simulink model "rubik_cube"  (R2022b)
settings: Solver=FixedStepDiscrete  StartTime=0.0  StopTime=10000.0  FixedStep=0.1  RelTol=1e-3
InitFcn:
  | mbd_s32k_consistency_checks(bdroot(gcs));
undefined symbols (not defined in the file or in its folder): LQFP
libraries: mbd_s32k1xx_ec_toolbox x5
settings Model: Creator=leona  LastModifiedBy=leona
settings SolverCC: ZeroCrossControl=DisableAll
settings DataIOCC: SaveOutput=off  SaveState=on  SaveTime=off
settings OptimizationCC: DefaultParameterBehavior=Inlined  EnhancedBackFolding=on  PassReuseOutputArgsAs=Individual arguments  ZeroExternalMemoryAtStartup=off  ZeroInternalMemoryAtStartup=off  OptimizeBlockOrder=speed  DifferentSizesBufferReuse=on  OptimizationCustomize=off  EfficientTunableParamExpr=on
settings DebuggingCC: InheritedTsInSrcMsg=none  SingleTaskRateTransMsg=error  ParameterTunabilityLossMsg=error  UnconnectedInputMsg=error  UnconnectedOutputMsg=error  UnconnectedLineMsg=error  UnknownTsInhSupMsg=error
settings HardwareCC: ProdBitPerPointer=32  ProdBitPerSizeT=32  ProdBitPerPtrDiffT=32  ProdLargestAtomicInteger=Long  ProdLargestAtomicFloat=Double  ProdWordSize=32  ProdHWDeviceType=ARM Compatible->ARM Cortex
settings ModelReferenceCC: ModelReferenceNumInstancesAllowed=Single
settings SFSimCC: MATLABDynamicMemAlloc=off
settings RTWCC: Description=Model Based Design Toolbox S32K1xx Code Generation Target  SystemTargetFile=mbd_s32k.tlc  MakeCommand=mbd_s32k_make_rtw COPY_MDLREF_INCLUDES=0  TemplateMakefile=mbd_s32k.tmf
settings CodeAppCC: ForceParamTrailComments=on  IgnoreCustomStorageClasses=off  OperatorAnnotations=on  SimulinkDataObjDesc=on  SFDataObjDesc=on  InsertBlockDesc=on
settings STFCustomTargetCC: TargetLangStandard=C99 (ISO)  MultiwordLength=256  ERTCustomFileBanners=on  SupportContinuousTime=off  SupportNonInlinedSFcns=off  RemoveResetFunc=on  MATLABClassNameForMDSCustomization=Simulink.SoftwareTarget.ERTCustomization  SystemTargetFile=mbd_s32k.tlc
settings ERTTargetCC: TargetLangStandard=C99 (ISO)  ParMdlRefBuildCompliant=off  CompOptLevelCompliant=off  ConcurrentExecutionCompliant=off  CombineOutputUpdateFcns=off  ModelStepFunctionPrototypeControlCompliant=off  CPPClassGenCompliant=off  UseToolchainInfoCompliant=off  InlinedParameterPlacement=NonHierarchical  ERTSrcFileBannerTemplate=mbd_ert_code_template.cgt  ERTHdrFileBannerTemplate=mbd_ert_code_template.cgt  ERTDataSrcFileTemplate=mbd_ert_code_template.cgt  ERTDataHdrFileTemplate=mbd_ert_code_template.cgt  ERTCustomFileTemplate=example_file_process.tlc

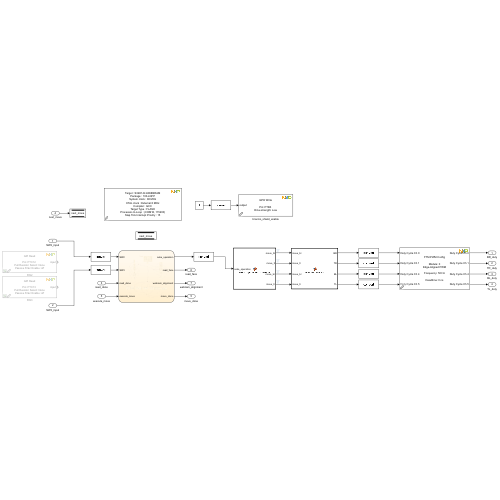
[thumbnail: Simulink's stored preview of the top-level diagram]
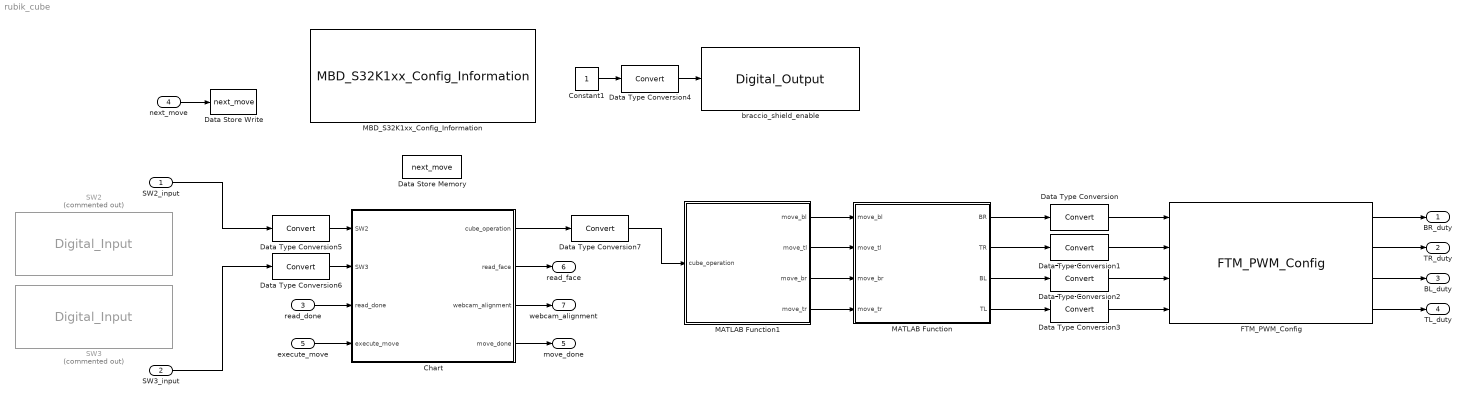
== system rubik_cube ==
  SW2_input : Inport
  SW3_input : Inport  Port=2
  read_done : Inport  Port=3
  next_move : Inport  Port=4
  execute_move : Inport  Port=5
  Chart : Stateflow chart  TreatAsAtomicUnit=on
  Constant1 : Constant
  Data Store Memory : DataStoreMemory  DataStoreName=next_move  WriteAfterWriteMsg=warning  InitialValue=uint8(zeros(1,2))  ShowAdditionalParam=off  OutDataTypeStr=uint8
  Data Store Write : DataStoreWrite  DataStoreName=next_move  IndexOptions=Index vector (dialog)  Indices=1  OutputSizes=1
  Data Type Conversion{,1..7} (8 alike) : DataTypeConversion  SaturateOnIntegerOverflow=off  RndMeth=Floor
  FTM_PWM_Config : mbd_s32k1xx_ec_toolbox/Motor Control Blocks/FTM Blocks/FTM_PWM_Config  ftmModule=0  ftmMode=Edge-Aligned PWM  ftmSourceClock=80 MHz  swcontrol_enable=off  chan0En=on  chan0Type=Independent  chan2En=off  chan2Type=Independent  chan4En=on  chan4Type=Independent  chan6En=off  chan6Type=Independent  ftmPwmUnits=Hz  outFrequency=50  ftmPeriod=25000  ftmPrescaler=Divide by 64  deadtimeUnits=Nanoseconds  deadtimeNs=0  deadtimeTicks=0  deadtimePrescaler=Divide by 1  dutyCycleCh0=0.03  dutyCycleCh1=0.125  dutyCycleCh2=0.025  dutyCycleCh3=0.025  dutyCycleCh4=0.025  dutyCycleCh5=0.025  dutyCycleCh6=0.25  dutyCycleCh7=0.25  dutyCycleSim=on  startAfterInit=on  showAdvOpt=on  pinFtmCh0=PTD15: [FTM0_CH0 | FTM Channel]  pinFtmCh1=PTD16: [FTM0_CH1 | FTM Channel]  pinPolCh0=Active High  pinPolCh1=Active High  outputComplem0=Main duplicated  outputLevel0=Low  outputLevel1=Low  pinFtmCh2=PTB14: [FTM0_CH2 | FTM Channel]  pinFtmCh3=PTC3: [FTM0_CH3 | FTM Channel]  pinPolCh2=Active High  pinPolCh3=Active High  outputComplem2=Main duplicated  outputLevel2=Low  outputLevel3=Low  pinFtmCh4=PTB4: [FTM0_CH4 | FTM Channel]  pinFtmCh5=PTB5: [FTM0_CH5 | FTM Channel]  pinPolCh4=Active High  pinPolCh5=Active High  outputComplem4=Main duplicated  outputLevel4=Low  outputLevel5=Low  pinFtmCh6=PTE8: [FTM0_CH6 | FTM Channel]  pinFtmCh7=None  pinPolCh6=Active High  pinPolCh7=Active High  outputComplem6=Main duplicated  outputLevel6=Low  outputLevel7=Low  initTrigger=off  chTrigger0=off  chTrigger1=off  chTrigger2=off  chTrigger3=off  chTrigger4=off  chTrigger5=off  chTrigger6=off  chTrigger7=off  mcuTargetUpdate=on  pwmSyncTrg=Software trigger  pwmSyncHwRouting=TRGMUX_FTM7  pwmSyncTrg0=off  pwmSyncTrg1=off  pwmSyncTrg2=off  pwmSyncAutoClear=on  pwmSyncMinLoad=on  pwmSyncMaxLoad=on  pwmSyncInvert=System Clock  pwmSyncOutControl=System Clock  pwmSyncOutMask=System Clock  pwmSyncCounterInitial=System Clock  pwmSyncPoints=Update now  reloadEnable=off  reloadPriority=15  reloadHalfCycle=off  reloadHCR=0  reloadFrequency=0  chnMatch0=off  chnMatch1=off  chnMatch2=off  chnMatch3=off  chnMatch4=off  chnMatch5=off  chnMatch6=off  chnMatch7=off  pwmFaultProtection=off  pwmFaultInterrupt=off  pwmFaultClearing=Fault control disabled  pwmFaultPinState=Safe Value  pwmFaultFilterValue=0  pwmFaultPriority=15  fault_disen_0=off  fault_filter_0=off  fault_polarity_0=Active High  fault_disen_1=off  fault_filter_1=off  fault_polarity_1=Active high  fault_disen_2=off  fault_filter_2=off  fault_polarity_2=Active high  fault_disen_3=off  fault_filter_3=off  fault_polarity_3=Active high  fault_pin_0=None  fault_pin_1=None  fault_pin_2=None  fault_pin_3=None
  MATLAB Function : MATLAB Function  TreatAsAtomicUnit=on
  MATLAB Function1 : MATLAB Function  TreatAsAtomicUnit=on
  MBD_S32K1xx_Config_Information : mbd_s32k1xx_ec_toolbox/MBD_S32K1xx_Config_Information  mbdt_ver=0  disp_str=|  config_params=[]  mcu_target_name=S32K144  mcu_target_package=100-LQFP  mcu_target_sram_size=48KB  mcu_system_clock_freq=80  mcu_xtal_freq=External 8  mcu_steptick_timer=LPIT Channel 0  mcu_steptick_prio=15  ds_import_enable=on  target_compiler=GCC  target_memory=FLASH  gcc_target_compile_opts=-mthumb -mfloat-abi=hard -mfpu=fpv4-sp-d16 -O1 -g -gstrict-dwarf  gcc_target_assemble_opts=-mthumb -mfloat-abi=hard -mfpu=fpv4-sp-d16 -g  gcc_target_link_opts=-mthumb -mfloat-abi=hard -mfpu=fpv4-sp-d16  gcc_target_default_lcf=on  gcc_target_user_lcf=S32K144_48_flash.ld  ghs_target_compile_opts=-cpu=cortexm4f -thumb -fpu=vfpv4_d16 -fsingle -Ogeneral -Wundef -Wimplicit-int -Wshadow -Wtrigraphs --no_commons --gnu_asm -gnu99 -gdwarf-2 -G  ghs_target_assemble_opts=-cpu=cortexm4f -fpu=vfpv4_d16  ghs_target_link_opts=-cpu=cortexm4f -thumb -fpu=vfpv4_d16  ghs_target_default_lcf=on  ghs_target_user_lcf=S32K144_48_flash.ld  iar_target_compile_opts=--cpu=Cortex-M4F --thumb --fpu=VFPv4_sp -Ol -e --debug --dlib_config normal  iar_target_assemble_opts=--cpu Cortex-M4F --thumb --fpu VFPv4_sp  iar_target_link_opts=--no_exceptions --vfe --inline  iar_target_default_lcf=on  iar_target_user_lcf=S32K144_48_flash.icf  pil_download_enable=on  rbl_download_enable=on  rbl_start_delay=5000  rbl_download_interface=OpenSDA  rbl_restart_request=off  rbl_com_port=Custom  rbl_com_port_custom=COM18  pil_download_rate=115200  pil_download_rate_custom=115200  pil_opensda_drive=F: EVB-S32K144  pil_opensda_drive_custom=D  jtag_interface=OpenSDA Embedded Debug  jlink_default_path=on  jlink_user_path=C:\Program Files\SEGGER\JLink\  pil_uart_instance=1  pil_uart_rx=PTC6: [LPUART1_RX | Receive]  pil_uart_tx=PTC7: [LPUART1_TX | Transmit]  FTM_PWM_PcrCheckEnDis=on  FTM_Input_Edge_Inputs_PcrCheckEnDis=on  FTM_Dual_Edge_Inputs_PcrCheckEnDis=on  FTM_Quadrature_Inputs_PcrCheckEnDis=on  FTM_Hall_Sensor_Inputs_PcrCheckEnDis=on  LPTMR_PcrCheckEnDis=on  PIT_PcrCheckEnDis=on  RTC_PcrCheckEnDis=on  FlexCAN_PcrCheckEnDis=on  LIN_PcrCheckEnDis=on  FlexIO_PcrCheckEnDis=on  LPI2C_PcrCheckEnDis=on  LPSPI_PcrCheckEnDis=on  LPUART_PcrCheckEnDis=on  CMP_PcrCheckEnDis=on  GPIO_OutputPcrCheckEnDis=on  GPIO_InputPcrCheckEnDis=on  SBC_PcrCheckEnDis=on  BMS_PcrCheckEnDis=on  AMMCLIB_PcrCheckEnDis=on  FM_PcrCheckEnDis=on  Profile_PcrCheckEnDis=on  ConfigParams_PcrCheckEnDis=on  ModelRef_PcrCheckEnDis=on  PDB0_PcrCheckEnDis=on  CSEc_PcrCheckEnDis=on  eDMA_PcrCheckEnDis=on  FLASH_PcrCheckEnDis=on  ADC_PcrCheckEnDis=on  WDOG_PcrCheckEnDis=on
      | Target : S32K144-64KB_SRAM
      | Package : 100-pin
      | System clock : 80 MHz
      | XTAL clock : External 8 MHz
      | Compiler : IAR
      | Target Type : FLASH
      | Download Code after build : off
      | Step Tick Interrupt Priority : 15
  SW2 : mbd_s32k1xx_ec_toolbox/GPIO Blocks/Digital_Input  Commented=on  gpio_pin=PTC12: [PTC12 | Port C I/O]  pull_resistor=None  passive_filter=off
  SW3 : mbd_s32k1xx_ec_toolbox/GPIO Blocks/Digital_Input  Commented=on  gpio_pin=PTC13: [PTC13 | Port C I/O]  pull_resistor=None  passive_filter=off
  braccio_shield_enable : mbd_s32k1xx_ec_toolbox/GPIO Blocks/Digital_Output  gpio_pin=PTB3: [PTB3 | Port B I/O]  init_val=Low  drive_strength=Low
  BR_duty : Outport
  TR_duty : Outport  Port=2
  BL_duty : Outport  Port=3
  TL_duty : Outport  Port=4
  move_done : Outport  Port=5
  read_face : Outport  Port=6
  webcam_alignment : Outport  Port=7
  wires:
  Data Type Conversion2/1 -> FTM_PWM_Config/3
  MATLAB Function1/3(move_br) -> MATLAB Function/3(move_br)
  FTM_PWM_Config/1 -> BR_duty/1
  MATLAB Function/4(TL) -> Data Type Conversion3/1
  FTM_PWM_Config/2 -> TR_duty/1
  Data Type Conversion5/1 -> Chart/1(SW2)
  Data Type Conversion4/1 -> braccio_shield_enable/1
  MATLAB Function/3(BL) -> Data Type Conversion2/1
  Chart/1(cube_operation) -> Data Type Conversion7/1
  Constant1/1 -> Data Type Conversion4/1
  MATLAB Function/1(BR) -> Data Type Conversion/1
  MATLAB Function1/1(move_bl) -> MATLAB Function/1(move_bl)
  FTM_PWM_Config/4 -> TL_duty/1
  Data Type Conversion7/1 -> MATLAB Function1/1(cube_operation)
  FTM_PWM_Config/3 -> BL_duty/1
  Data Type Conversion3/1 -> FTM_PWM_Config/4
  MATLAB Function/2(TR) -> Data Type Conversion1/1
  Data Type Conversion6/1 -> Chart/2(SW3)
  Data Type Conversion1/1 -> FTM_PWM_Config/2
  MATLAB Function1/4(move_tr) -> MATLAB Function/4(move_tr)
  Data Type Conversion/1 -> FTM_PWM_Config/1
  MATLAB Function1/2(move_tl) -> MATLAB Function/2(move_tl)
  SW2_input/1 -> Data Type Conversion5/1
  SW3_input/1 -> Data Type Conversion6/1
  Chart/2(read_face) -> read_face/1
  Chart/3(webcam_alignment) -> webcam_alignment/1
  Chart/4(move_done) -> move_done/1
  read_done/1 -> Chart/3(read_done)
  execute_move/1 -> Chart/4(execute_move)
  next_move/1 -> Data Store Write/1

== matlab function rubik_cube/MATLAB Function1 ==
  data: cube_operation input; move_bl output; move_tl output; move_br output; move_tr output
function [move_bl, move_tl, move_br, move_tr] = cube_operation_decoder(cube_operation)
% This function takes as input the code for a cube operation and converts
% it as positions of the 4 servo motors. The operations must be a 4 digit
% unsigned integer, encoded as follows:
%   - first digit [0, 1]: open/close left grip;
%   - second digit [0, 1]: open/close right grip;
%   - third digit [0, 1, 2]: set left arm to 90/0/180 degrees
%   - fourth digit [0, 1, 2]: set right arm to 90/0/180 degress

x1 = int32(mod(cube_operation/1000, 10));
x2 = int32(mod(cube_operation/100, 10));
x3 = int32(mod(cube_operation/10, 10));
x4 = int32(mod(cube_operation, 10));

move_tl = x1;
move_tr = x2;
move_bl = x3;
move_br = x4;

== matlab function rubik_cube/MATLAB Function ==
  data: BR output; TR output; move_bl input; BL output; move_tl input; move_br input; move_tr input; TL output
function [BR, TR, BL, TL] = actuate_servos(move_bl, move_tl, move_br, move_tr)
% This function takes as input as specific number associated to a movement
% of the 4 servo motors (BL = Bottom Left, TL = Top Left, BR = Bottom Right,
% TR = Top Right) and it gives as output the 4 relative duty cycles needed to
% obtain that movement. 

min_duty = 0.025;
max_duty = 0.125;

duty_0_deg = min_duty;
duty_grip_open = min_duty + (max_duty-min_duty)/3;
duty_grip_closed = min_duty + (max_duty-min_duty)/9; 
duty_90_deg = min_duty + (max_duty-min_duty)/2;
duty_180_deg = max_duty;

switch (move_tl)
    case 0                  % Open left grip
        TL = duty_grip_open;
    case 1                  % Close left grip
        TL = duty_grip_closed;
    otherwise               % Open left grip
        TL = duty_grip_open;
end

switch (move_tr)
    case 0                  % Open right grip
        TR = duty_grip_open;
    case 1                  % Close right grip
        TR = duty_grip_closed;
    otherwise               % Open right grip
        TR = duty_grip_open;
end

switch (move_bl)
    case 0                  % Left arm straight
        BL = duty_90_deg;
    case 1                  % Left arm at 90° clockwise
        BL = duty_0_deg;
    case 2                  % Left arm at 90° counter-clockwise
        BL = duty_180_deg;
    otherwise
        BL = duty_90_deg;
end

switch (move_br)
    case 0                  % Right arm straight
        BR = duty_90_deg;
    case 1                  % Right arm at 90° clockwise
        BR = duty_0_deg;
    case 2                  % Right arm at 90° counter-clockwise
        BR = duty_180_deg;
    otherwise
        BR = duty_90_deg;
end

% Update current position of the motors
BL_last_move = move_bl;
TL_last_move = move_tl;
BR_last_move = move_br;
TR_last_move = move_tr;

== stateflow chart rubik_cube/Chart ==
  state read_cube
    en:
    webcam_alignment = 0;
    SW3_status = SW3;
    du:
    SW3_status = SW3;
    % Clear cube colors
    %cube = zeros(3, 3, 6);
    %read red
    %LTm
    %read blue
    %LTm
    %read orange
    %LTm
    %read green
    %RTm
    %LTm
    %read white
    %RTmm
    %LTmm
    %read yellow
    %RTm
    %LTm
    %RTp
    state read_red
      en:
      read_face = 1;
    state wait_red
      en:
      read_face = 0;
    state fase1
      en:
      cube_operation=1000
    state fase2
      en:
      cube_operation=1010
    state fase3
      en:
      cube_operation=1110
    state fase4
      en:
      cube_operation=0110
    state fase5
      en:
      cube_operation=0100
    state fase6
      en:
      cube_operation=1100
    state fase12
      en:
      cube_operation=1100
    state fase11
      en:
      cube_operation=0100
    state fase10
      en:
      cube_operation=0110
    state fase9
      en:
      cube_operation=1110
    state fase8
      en:
      cube_operation=1010
    state fase7
      en:
      cube_operation=1000
    state wait_blue
      en:
      read_face = 0;
    state read_blue
      en:
      read_face = 1;
    state read_orange
      en:
      read_face=1;
    state wait_orange
      en:
      read_face=0;
    state fase13
      en:
      cube_operation=1000
    state fase14
      en:
      cube_operation=1010
    state fase15
      en:
      cube_operation=1110
    state fase16
      en:
      cube_operation=0110
    state fase17
      en:
      cube_operation=0100
    state fase18
      en:
      cube_operation=1100
    state fase24
      en:
      cube_operation=1100
    state fase23
      en:
      cube_operation=1000
    state fase22
      en:
      cube_operation=1001
    state fase21
      en:
      cube_operation=1101
    state fase20
      en:
      cube_operation=0101
    state fase19
      en:
      cube_operation=0100
    state wait_green
      en:
      read_face=0;
    state read_green
      en:
      read_face=1;
    state fase27
      en:
      cube_operation=1110
    state fase25
      en:
      cube_operation=1000
    state fase26
      en:
      cube_operation=1010
    state fase28
      en:
      cube_operation=0110
    state fase29
      en:
      cube_operation=0100
    state fase30
      en:
      cube_operation=1100
    state read_white
      en:
      read_face=1;
    state wait_white
      en:
      read_face=0;
    state fase35
      en:
      cube_operation=1000
    state fase37
      en:
      cube_operation=0100
    state fase36
      en:
      cube_operation=1100
    state fase34
      en:
      cube_operation=1001
    state fase33
      en:
      cube_operation=1101
    state fase32
      en:
      cube_operation=0101
    state fase31
      en:
      cube_operation=0100
    state fase38
      en:
      cube_operation=0101
    state fase39
      en:
      cube_operation=1101
    state fase40
      en:
      cube_operation=1001
    state fase41
      en:
      cube_operation=1000
    state fase42
      en:
      cube_operation=1100
    state fase43
      en:
      cube_operation=1000
    state fase44
      en:
      cube_operation=1010
    state fase51
      en:
      cube_operation=1110
    state fase50
      en:
      cube_operation=1010
    state fase49
      en:
      cube_operation=1000
    state fase48
      en:
      cube_operation=1100
    state fase47
      en:
      cube_operation=0100
    state fase46
      en:
      cube_operation=0110
    state fase45
      en:
      cube_operation=1110
    state read_yellow
      en:
      read_face=1;
    state wait_yellow
      en:
      read_face=0;
    state fase55
      en:
      cube_operation=0100
    state fase56
      en:
      cube_operation=0101
    state fase57
      en:
      cube_operation=1101
    state fase52
      en:
      cube_operation=0110
    state fase54
      en:
      cube_operation=1100
    state fase53
      en:
      cube_operation=0100
    state fase58
      en:
      cube_operation=1001
    state fase63
      en:
      cube_operation=1110
    state fase64
      en:
      cube_operation=0110
    state fase62
      en:
      cube_operation=1010
    state fase61
      en:
      cube_operation=1000
    state fase60
      en:
      cube_operation=1100
    state fase59
      en:
      cube_operation=1000
    state fase65
      en:
      cube_operation=0100
    state fase66
      en:
      cube_operation=1100
    state fase67
      en:
      cube_operation=1000
    state fase68
      en:
      cube_operation=1001
    state fase69
      en:
      cube_operation=1101
    state fase70
      en:
      cube_operation=0101
    state fase71
      en:
      cube_operation=0100
    state fase72
      en:
      cube_operation=1100
    (default) -> read_red
    wait_red -> read_red [order 2] : [read_done==2]
    read_red -> wait_red
    wait_red -> read_cube.fase1 [order 1] : [read_done==1]
    read_cube.fase1 -> read_cube.fase2 : [SW3 == 1]
    read_cube.fase2 -> read_cube.fase3 : [after(delay_ms, msec)]
    read_cube.fase3 -> read_cube.fase4 : [after(delay_ms, msec)]
    read_cube.fase4 -> read_cube.fase5 : [after(delay_ms, msec)]
    read_cube.fase5 -> read_cube.fase6 : [after(delay_ms, msec)]
    read_cube.fase6 -> read_blue : [after(delay_ms, msec)]
    wait_blue -> read_blue [order 2] : [read_done==2]
    read_blue -> wait_blue
    read_cube.fase11 -> read_cube.fase12 : [after(delay_ms, msec)]
    read_cube.fase10 -> read_cube.fase11 : [after(delay_ms, msec)]
    read_cube.fase9 -> read_cube.fase10 : [after(delay_ms, msec)]
    read_cube.fase8 -> read_cube.fase9 : [after(delay_ms, msec)]
    read_cube.fase7 -> read_cube.fase8 : [SW3 == 1]
    wait_blue -> read_cube.fase7 [order 1] : [read_done==1]
    read_cube.fase12 -> read_orange : [after(delay_ms, msec)]
    wait_orange -> read_orange [order 1] : [read_done==2]
    read_orange -> wait_orange
    wait_orange -> read_cube.fase13 [order 2] : [read_done==1]
    read_cube.fase13 -> read_cube.fase14 : [SW3 == 1]
    read_cube.fase14 -> read_cube.fase15 : [after(delay_ms, msec)]
    read_cube.fase15 -> read_cube.fase16 : [after(delay_ms, msec)]
    read_cube.fase16 -> fase17 : [after(delay_ms, msec)]
    fase17 -> fase18 : [after(delay_ms, msec)]
    fase18 -> read_green : [after(delay_ms, msec)]
    read_green -> wait_green
    fase23 -> fase24 : [after(delay_ms, msec)]
    fase22 -> fase23 : [after(delay_ms, msec)]
    fase21 -> fase22 : [after(delay_ms, msec)]
    fase20 -> fase21 : [after(delay_ms, msec)]
    fase19 -> fase20 : [SW3 == 1]
    wait_green -> fase19 [order 1] : [read_done==1]
    wait_green -> read_green [order 2] : [read_done==2]
    fase24 -> fase25 : [after(delay_ms, msec)]
    read_white -> wait_white
    fase26 -> fase27 : [after(delay_ms, msec)]
    fase27 -> fase28 : [after(delay_ms, msec)]
    fase25 -> fase26 : [after(delay_ms, msec)]
    fase28 -> fase29 : [after(delay_ms, msec)]
    fase29 -> fase30 : [after(delay_ms, msec)]
    wait_white -> read_white [order 2] : [read_done==2]
    fase30 -> read_white : [after(delay_ms, msec)]
    wait_white -> fase31 [order 1] : [read_done==1]
    fase35 -> fase36 : [after(delay_ms, msec)]
    fase34 -> fase35 : [[after(delay_ms, msec)]]
    fase36 -> fase37 : [after(delay_ms, msec)]
    fase33 -> fase34 : [after(delay_ms, msec)]
    fase32 -> fase33 : [after(delay_ms, msec)]
    fase31 -> fase32 : [SW3 == 1]
    fase37 -> fase38 : [after(delay_ms, msec)]
    fase39 -> fase40 : [after(delay_ms, msec)]
    fase38 -> fase39 : [after(delay_ms, msec)]
    fase40 -> fase41 : [after(delay_ms, msec)]
    fase41 -> fase42 : [after(delay_ms, msec)]
    fase42 -> fase43 : [after(delay_ms, msec)]
    fase43 -> fase44 : [after(delay_ms, msec)]
    fase44 -> fase45 : [after(delay_ms, msec)]
    fase49 -> fase50 : [after(delay_ms, msec)]
    fase48 -> fase49 : [after(delay_ms, msec)]
    fase46 -> fase47 : [after(delay_ms, msec)]
    fase45 -> fase46 : [after(delay_ms, msec)]
    fase50 -> fase51 : [after(delay_ms, msec)]
    fase47 -> fase48 : [after(delay_ms, msec)]
    fase51 -> fase52 : [after(delay_ms, msec)]
    fase56 -> fase57 : [after(delay_ms, msec)]
    fase54 -> read_yellow : [after(delay_ms, msec)]
    fase55 -> fase56 : [SW3 == 1]
    read_yellow -> wait_yellow
    wait_yellow -> fase55 [order 2] : [read_done==1]
    fase52 -> fase53 : [after(delay_ms, msec)]
    fase53 -> fase54 : [after(delay_ms, msec)]
    wait_yellow -> read_yellow [order 1] : [read_done==2]
    fase57 -> fase58 : [after(delay_ms, msec)]
    fase62 -> fase63 : [after(delay_ms, msec)]
    fase61 -> fase62 : [after(delay_ms, msec)]
    fase60 -> fase61 : [after(delay_ms, msec)]
    fase59 -> fase60 : [after(delay_ms, msec)]
    fase63 -> fase64 : [after(delay_ms, msec)]
    fase58 -> fase59 : [after(delay_ms, msec)]
    fase64 -> fase65 : [after(delay_ms, msec)]
    fase65 -> fase66 : [after(delay_ms, msec)]
    fase66 -> fase67 : [after(delay_ms, msec)]
    fase67 -> fase68 : [after(delay_ms, msec)]
    fase68 -> fase69 : [after(delay_ms, msec)]
    fase69 -> fase70 : [after(delay_ms, msec)]
    fase70 -> fase71 : [after(delay_ms, msec)]
    fase71 -> fase72 : [after(delay_ms, msec)]
  state webcam_alignment
    en:
    SW2_status = SW2;
    SW3_status = SW3;
    cube_operation=1100;
    webcam_alignment = 1;
    du:
    SW2_status=SW2;
    SW3_status=SW3;
  state wait_cube
    en:
    SW2_status = SW2;
    cube_operation=0100;
    move_done = 1;
    du:
    SW2_status=SW2;
  state D
    en:
    %LMp
    state fase1 %LMp
      en:
      cube_operation=0100;
    state fase2
      en:
      cube_operation=0110;
    state fase3
      en:
      cube_operation=1110;
    state fase4
      en:
      cube_operation=1100;
    (default) -> fase1 %LMp
    fase1 %LMp -> D.fase2 : [after(delay_ms,msec)]
    D.fase2 -> D.fase3 : [after(delay_ms,msec)]
    D.fase3 -> D.fase4 : [after(delay_ms,msec)]
  state Fi
    en:
    %LTpp
    %RMm
    state fase1
      en:
      cube_operation=0100;
    state fase1bis
      en:
      cube_operation=0110;
    state fase2
      en:
      cube_operation=1110;
    state fase4
      en:
      cube_operation=1120;
    state fase3bis
      en:
      cube_operation=1020;
    state fase3
      en:
      cube_operation=1010;
    state fase5bis
      en:
      cube_operation=0100;
    state fase6
      en:
      cube_operation=1100
    state fase5
      en:
      cube_operation=0120;
    state fase8bis
      en:
      cube_operation=1000;
    state fase8
      en:
      cube_operation=1001;
    state fase7 %RMm
      en:
      cube_operation=1101;
    state fase9
      en:
      cube_operation=1100;
    (default) -> Fi.fase1
    Fi.fase1 -> Fi.fase1bis : [after(delay_ms,msec)]
    Fi.fase1bis -> Fi.fase2 : [after(delay_ms,msec)]
    Fi.fase2 -> Fi.fase3 : [after(delay_ms,msec)]
    Fi.fase3bis -> Fi.fase4 : [after(delay_ms,msec)]
    Fi.fase3 -> Fi.fase3bis : [after(delay_ms,msec)]
    Fi.fase4 -> Fi.fase5 : [after(delay_ms,msec)]
    Fi.fase5bis -> Fi.fase6 : [after(delay_ms,msec)]
    Fi.fase5 -> Fi.fase5bis : [after(delay_ms,msec)]
    Fi.fase6 -> fase7 %RMm : [after(delay_ms,msec)]
    fase7 %RMm -> Fi.fase8 : [after(delay_ms,msec)]
    Fi.fase8 -> fase8bis : [after(delay_ms,msec)]
    fase8bis -> Fi.fase9 : [after(delay_ms,msec)]
  state solve_cube
    en:
    move_done = 1;
    ex:
    move_done = 0;
  state D2
    en:
    %LMpp
    state fase1 %LMpp
      en:
      cube_operation=0100;
    state fase2
      en:
      cube_operation=0110;
    state fase4
      en:
      cube_operation=1120;
    state fase3
      en:
      cube_operation=1110;
    state fase6
      en:
      cube_operation=0100;
    state fase5
      en:
      cube_operation=0120;
    state fase7
      en:
      cube_operation=1100;
    (default) -> fase1 %LMpp
    fase1 %LMpp -> D2.fase2 : [after(delay_ms,msec)]
    D2.fase2 -> D2.fase3 : [after(delay_ms,msec)]
    D2.fase3 -> D2.fase4 : [after(delay_ms,msec)]
    D2.fase4 -> D2.fase5 : [after(delay_ms,msec)]
    D2.fase5 -> D2.fase6 : [after(delay_ms,msec)]
    D2.fase6 -> D2.fase7 : [after(delay_ms,msec)]
  state F
    en:
    %LTpp
    %RMp
    state fase1
      en:
      cube_operation=0100;
    state fase1bis
      en:
      cube_operation=0110;
    state fase2
      en:
      cube_operation=1110;
    state fase4
      en:
      cube_operation=1120;
    state fase3bis
      en:
      cube_operation=1020;
    state fase3
      en:
      cube_operation=1010;
    state fase5bis
      en:
      cube_operation=0100;
    state fase6
      en:
      cube_operation=1100
    state fase5
      en:
      cube_operation=0120;
    state fase8
      en:
      cube_operation=1101;
    state fase7bis
      en:
      cube_operation=1001;
    state fase7 %RMp
      en:
      cube_operation=1000;
    state fase9
      en:
      cube_operation=1100;
    F.fase1 -> F.fase1bis : [after(delay_ms,msec)]
    F.fase1bis -> F.fase2 : [after(delay_ms,msec)]
    (default) -> F.fase1
    F.fase2 -> F.fase3 : [after(delay_ms,msec)]
    F.fase3bis -> F.fase4 : [after(delay_ms,msec)]
    F.fase3 -> F.fase3bis : [after(delay_ms,msec)]
    F.fase4 -> F.fase5 : [after(delay_ms,msec)]
    F.fase5bis -> F.fase6 : [after(delay_ms,msec)]
    F.fase5 -> F.fase5bis : [after(delay_ms,msec)]
    F.fase6 -> fase7 %RMp : [after(delay_ms,msec)]
    fase7 %RMp -> F.fase7bis : [after(delay_ms,msec)]
    F.fase7bis -> F.fase8 : [after(delay_ms,msec)]
    F.fase8 -> F.fase9 : [after(delay_ms,msec)]
  state Di
    en:
    %LMm
    state fase1 %LMm
      en:
      cube_operation=1110;
    state fase2
      en:
      cube_operation=0110;
    state fase3
      en:
      cube_operation=0100;
    state fase4
      en:
      cube_operation=1100;
    (default) -> fase1 %LMm
    fase1 %LMm -> Di.fase2 : [after(delay_ms,msec)]
    Di.fase2 -> Di.fase3 : [after(delay_ms,msec)]
    Di.fase3 -> Di.fase4 : [after(delay_ms,msec)]
  state F2
    en:
    %LTpp
    %RMpp
    state fase1
      en:
      cube_operation=0100;
    state fase1bis
      en:
      cube_operation=0110;
    state fase2
      en:
      cube_operation=1110;
    state fase4
      en:
      cube_operation=1120;
    state fase3bis
      en:
      cube_operation=1020;
    state fase3
      en:
      cube_operation=1010;
    state fase5bis
      en:
      cube_operation=0100;
    state fase6
      en:
      cube_operation=1100
    state fase5
      en:
      cube_operation=0120;
    state fase12 %RMpp
      en:
      cube_operation=1000;
    state fase7bis
      en:
      cube_operation=1001;
    state fase9
      en:
      cube_operation=1102;
    state fase8
      en:
      cube_operation=1101;
    state fase10
      en:
      cube_operation=1002;
    state fase11
      en:
      cube_operation=1100;
    state fase10bis
      en:
      cube_operation=1000;
    F2.fase1 -> F2.fase1bis : [after(delay_ms,msec)]
    F2.fase1bis -> F2.fase2 : [after(delay_ms,msec)]
    (default) -> F2.fase1
    F2.fase2 -> F2.fase3 : [after(delay_ms,msec)]
    F2.fase3bis -> F2.fase4 : [after(delay_ms,msec)]
    F2.fase3 -> F2.fase3bis : [after(delay_ms,msec)]
    F2.fase4 -> F2.fase5 : [after(delay_ms,msec)]
    F2.fase5bis -> F2.fase6 : [after(delay_ms,msec)]
    F2.fase5 -> F2.fase5bis : [after(delay_ms,msec)]
    F2.fase6 -> fase12 %RMpp : [after(delay_ms,msec)]
    fase12 %RMpp -> F2.fase7bis : [after(delay_ms,msec)]
    F2.fase7bis -> F2.fase8 : [after(delay_ms,msec)]
    F2.fase9 -> F2.fase10 : [after(delay_ms,msec)]
    F2.fase8 -> F2.fase9 : [after(delay_ms,msec)]
    F2.fase10 -> fase10bis : [after(delay_ms,msec)]
    fase10bis -> F2.fase11 : [after(delay_ms,msec)]
  state B
    en:
    %RMp
    state fase1 %RMp
      en:
      cube_operation=1000;
    state fase2
      en:
      cube_operation=1001;
    state fase3
      en:
      cube_operation=1101;
    state fase4
      en:
      cube_operation=1100;
    (default) -> fase1 %RMp
    fase1 %RMp -> B.fase2 : [after(delay_ms,msec)]
    B.fase2 -> B.fase3 : [after(delay_ms,msec)]
    B.fase3 -> B.fase4 : [after(delay_ms,msec)]
  state U
    %RTpp
    %LMp
    state fase1 %RTpp
      en:
      cube_operation=1000;
    state fase2
      en:
      cube_operation=1001;
    state fase3
      en:
      cube_operation=1101;
    state fase6
      en:
      cube_operation=1102;
    state fase5
      en:
      cube_operation=0102;
    state fase4
      en:
      cube_operation=0101;
    state fase8
      en:
      cube_operation=1000;
    state fase9
      en:
      cube_operation=1100;
    state fase7
      en:
      cube_operation=1002;
    state fase12
      en:
      cube_operation=1110;
    state fase11
      en:
      cube_operation=0110;
    state fase10 %LMp
      en:
      cube_operation=0100;
    state fase13
      en:
      cube_operation=1100;
    (default) -> U.fase1 %RTpp
    U.fase2 -> U.fase3 : [after(delay_ms,msec)]
    U.fase1 %RTpp -> U.fase2 : [after(delay_ms,msec)]
    U.fase3 -> U.fase4 : [after(delay_ms,msec)]
    U.fase4 -> U.fase5 : [after(delay_ms,msec)]
    U.fase5 -> U.fase6 : [after(delay_ms,msec)]
    U.fase6 -> U.fase7 : [after(delay_ms,msec)]
    U.fase7 -> U.fase8 : [after(delay_ms,msec)]
    U.fase8 -> U.fase9 : [after(delay_ms,msec)]
    U.fase9 -> fase10 %LMp : [after(delay_ms,msec)]
    U.fase11 -> U.fase12 : [after(delay_ms,msec)]
    fase10 %LMp -> U.fase11 : [after(delay_ms,msec)]
    U.fase12 -> U.fase13 : [after(delay_ms,msec)]
  state B2
    en:
    %RMpp
    state fase1 %RMpp
      en:
      cube_operation=1000;
    state fase2
      en:
      cube_operation=1001;
    state fase4
      en:
      cube_operation=1102;
    state fase3
      en:
      cube_operation=1101;
    state fase5
      en:
      cube_operation=1002;
    state fase6
      en:
      cube_operation=1000;
    state fase7
      en:
      cube_operation=1100;
    (default) -> fase1 %RMpp
    fase1 %RMpp -> B2.fase2 : [after(delay_ms,msec)]
    B2.fase2 -> B2.fase3 : [after(delay_ms,msec)]
    B2.fase3 -> B2.fase4 : [after(delay_ms,msec)]
    B2.fase4 -> B2.fase5 : [after(delay_ms,msec)]
    B2.fase5 -> B2.fase6 : [after(delay_ms,msec)]
    B2.fase6 -> B2.fase7 : [after(delay_ms,msec)]
  state U2
    %RTpp
    %LMpp
    state fase1 %RTpp
      en:
      cube_operation=1000;
    state fase2
      en:
      cube_operation=1001;
    state fase3
      en:
      cube_operation=1101;
    state fase6
      en:
      cube_operation=1102;
    state fase5
      en:
      cube_operation=0102;
    state fase4
      en:
      cube_operation=0101;
    state fase8
      en:
      cube_operation=1000;
    state fase9
      en:
      cube_operation=1100;
    state fase7
      en:
      cube_operation=1002;
    state fase11
      en:
      cube_operation=0110;
    state fase10 %LMpp
      en:
      cube_operation=0100;
    state fase12
      en:
      cube_operation=1110;
    state fase13
      en:
      cube_operation=1120;
    state fase14
      en:
      cube_operation=0120;
    state fase15
      en:
      cube_operation=0100;
    state fase16
      en:
      cube_operation=1100;
    (default) -> U2.fase1 %RTpp
    U2.fase2 -> U2.fase3 : [after(delay_ms,msec)]
    U2.fase1 %RTpp -> U2.fase2 : [after(delay_ms,msec)]
    U2.fase3 -> U2.fase4 : [after(delay_ms,msec)]
    U2.fase4 -> U2.fase5 : [after(delay_ms,msec)]
    U2.fase5 -> U2.fase6 : [after(delay_ms,msec)]
    U2.fase6 -> U2.fase7 : [after(delay_ms,msec)]
    U2.fase7 -> U2.fase8 : [after(delay_ms,msec)]
    U2.fase8 -> U2.fase9 : [after(delay_ms,msec)]
    U2.fase9 -> fase10 %LMpp : [after(delay_ms,msec)]
    U2.fase11 -> U2.fase12 : [after(delay_ms,msec)]
    fase10 %LMpp -> U2.fase11 : [after(delay_ms,msec)]
    U2.fase12 -> U2.fase13 : [after(delay_ms,msec)]
    U2.fase13 -> U2.fase14 : [after(delay_ms,msec)]
    U2.fase14 -> U2.fase15 : [after(delay_ms,msec)]
    U2.fase15 -> U2.fase16 : [after(delay_ms,msec)]
  state Bi
    en:
    %RMm
    state fase1 %RMm
      en:
      cube_operation=1101;
    state fase2
      en:
      cube_operation=1001;
    state fase3
      en:
      cube_operation=1000;
    state fase4
      en:
      cube_operation=1100;
    (default) -> fase1 %RMm
    fase1 %RMm -> Bi.fase2 : [after(delay_ms,msec)]
    Bi.fase2 -> Bi.fase3 : [after(delay_ms,msec)]
    Bi.fase3 -> Bi.fase4 : [after(delay_ms,msec)]
  state Ui
    %RTpp
    %LMm
    state fase1 %RTpp
      en:
      cube_operation=1000;
    state fase2
      en:
      cube_operation=1001;
    state fase3
      en:
      cube_operation=1101;
    state fase6
      en:
      cube_operation=1102;
    state fase5
      en:
      cube_operation=0102;
    state fase4
      en:
      cube_operation=0101;
    state fase8
      en:
      cube_operation=1000;
    state fase9
      en:
      cube_operation=1100;
    state fase7
      en:
      cube_operation=1002;
    state fase12
      en:
      cube_operation=0100;
    state fase11
      en:
      cube_operation=0110;
    state fase10 %LMm
      en:
      cube_operation=1110;
    state fase13
      en:
      cube_operation=1100;
    (default) -> Ui.fase1 %RTpp
    Ui.fase2 -> Ui.fase3 : [after(delay_ms,msec)]
    Ui.fase1 %RTpp -> Ui.fase2 : [after(delay_ms,msec)]
    Ui.fase3 -> Ui.fase4 : [after(delay_ms,msec)]
    Ui.fase4 -> Ui.fase5 : [after(delay_ms,msec)]
    Ui.fase5 -> Ui.fase6 : [after(delay_ms,msec)]
    Ui.fase6 -> Ui.fase7 : [after(delay_ms,msec)]
    Ui.fase7 -> Ui.fase8 : [after(delay_ms,msec)]
    Ui.fase8 -> Ui.fase9 : [after(delay_ms,msec)]
    Ui.fase9 -> fase10 %LMm : [after(delay_ms,msec)]
    Ui.fase11 -> Ui.fase12 : [after(delay_ms,msec)]
    fase10 %LMm -> Ui.fase11 : [after(delay_ms,msec)]
    Ui.fase12 -> Ui.fase13 : [after(delay_ms,msec)]
  state R
    en:
    %RTm
    %LMp
    state fase1
      en:
      cube_operation=0100;
    state fase2
      en:
      cube_operation=0101;
    state fase3
      en:
      cube_operation=1101;
    state fase6
      en:
      cube_operation=1100
    state fase5
      en:
      cube_operation=1000;
    state fase4
      en:
      cube_operation=1001;
    state fase7 %LMp
      en:
      cube_operation=0100;
    state fase8
      en:
      cube_operation=0110;
    state fase9
      en:
      cube_operation=1110;
    state fase10
      en:
      cube_operation=1100;
    (default) -> R.fase1
    R.fase2 -> R.fase3 : [after(delay_ms,msec)]
    R.fase1 -> R.fase2 : [after(delay_ms,msec)]
    R.fase3 -> R.fase4 : [after(delay_ms,msec)]
    R.fase5 -> R.fase6 : [after(delay_ms,msec)]
    R.fase4 -> R.fase5 : [after(delay_ms,msec)]
    R.fase6 -> R.fase7 %LMp : [after(delay_ms,msec)]
    R.fase7 %LMp -> R.fase8 : [after(delay_ms,msec)]
    R.fase9 -> R.fase10 : [after(delay_ms,msec)]
    R.fase8 -> R.fase9 : [after(delay_ms,msec)]
  state L
    en:
    %RTp
    %LMp
    state fase1
      en:
      cube_operation=1000;
    state fase2
      en:
      cube_operation=1001;
    state fase3
      en:
      cube_operation=1101;
    state fase6
      en:
      cube_operation=1100
    state fase5
      en:
      cube_operation=0100;
    state fase4
      en:
      cube_operation=0101;
    state fase7 %LMp
      en:
      cube_operation=0100;
    state fase8
      en:
      cube_operation=0110;
    state fase9
      en:
      cube_operation=1110;
    state fase10
      en:
      cube_operation=1100;
    (default) -> L.fase1
    L.fase2 -> L.fase3 : [after(delay_ms,msec)]
    L.fase1 -> L.fase2 : [after(delay_ms,msec)]
    L.fase3 -> L.fase4 : [after(delay_ms,msec)]
    L.fase5 -> L.fase6 : [after(delay_ms,msec)]
    L.fase4 -> L.fase5 : [after(delay_ms,msec)]
    L.fase6 -> L.fase7 %LMp : [after(delay_ms,msec)]
    L.fase7 %LMp -> L.fase8 : [after(delay_ms,msec)]
    L.fase9 -> L.fase10 : [after(delay_ms,msec)]
    L.fase8 -> L.fase9 : [after(delay_ms,msec)]
  state R2
    en:
    %RTm
    %LMpp
    state fase1
      en:
      cube_operation=0100;
    state fase2
      en:
      cube_operation=0101;
    state fase3
      en:
      cube_operation=1101;
    state fase4
      en:
      cube_operation=1001;
    state fase7 %LMpp
      en:
      cube_operation=0100;
    state fase6
      en:
      cube_operation=1100
    state fase8
      en:
      cube_operation=0110;
    state fase5
      en:
      cube_operation=1000;
    state fase9
      en:
      cube_operation=1110;
    state fase10
      en:
      cube_operation=1120;
    state fase11
      en:
      cube_operation=0120;
    state fase12
      en:
      cube_operation=0100;
    state fase13
      en:
      cube_operation=1100;
    R2.fase2 -> R2.fase3 : [after(delay_ms,msec)]
    R2.fase1 -> R2.fase2 : [after(delay_ms,msec)]
    R2.fase3 -> R2.fase4 : [after(delay_ms,msec)]
    (default) -> R2.fase1
    R2.fase4 -> R2.fase5 : [after(delay_ms,msec)]
    R2.fase7 %LMpp -> R2.fase8 : [after(delay_ms,msec)]
    R2.fase6 -> R2.fase7 %LMpp : [after(delay_ms,msec)]
    R2.fase5 -> R2.fase6 : [after(delay_ms,msec)]
    R2.fase8 -> R2.fase9 : [after(delay_ms,msec)]
    R2.fase10 -> R2.fase11 : [after(delay_ms,msec)]
    R2.fase9 -> R2.fase10 : [after(delay_ms,msec)]
    R2.fase11 -> R2.fase12 : [after(delay_ms,msec)]
    R2.fase12 -> R2.fase13 : [after(delay_ms,msec)]
  state L2
    en:
    %RTp
    %LMpp
    state fase1
      en:
      cube_operation=1000;
    state fase2
      en:
      cube_operation=1001;
    state fase3
      en:
      cube_operation=1101;
    state fase4
      en:
      cube_operation=0101;
    state fase7 %LMpp
      en:
      cube_operation=0100;
    state fase6
      en:
      cube_operation=1100
    state fase8
      en:
      cube_operation=0110;
    state fase5
      en:
      cube_operation=0100;
    state fase9
      en:
      cube_operation=1110;
    state fase10
      en:
      cube_operation=1120;
    state fase11
      en:
      cube_operation=0120;
    state fase12
      en:
      cube_operation=0100;
    state fase13
      en:
      cube_operation=1100;
    L2.fase2 -> L2.fase3 : [after(delay_ms,msec)]
    L2.fase1 -> L2.fase2 : [after(delay_ms,msec)]
    L2.fase3 -> L2.fase4 : [after(delay_ms,msec)]
    (default) -> L2.fase1
    L2.fase4 -> L2.fase5 : [after(delay_ms,msec)]
    L2.fase7 %LMpp -> L2.fase8 : [after(delay_ms,msec)]
    L2.fase6 -> L2.fase7 %LMpp : [after(delay_ms,msec)]
    L2.fase5 -> L2.fase6 : [after(delay_ms,msec)]
    L2.fase8 -> L2.fase9 : [after(delay_ms,msec)]
    L2.fase10 -> L2.fase11 : [after(delay_ms,msec)]
    L2.fase9 -> L2.fase10 : [after(delay_ms,msec)]
    L2.fase11 -> L2.fase12 : [after(delay_ms,msec)]
    L2.fase12 -> L2.fase13 : [after(delay_ms,msec)]
  state Ri
    en:
    %RTm
    %LMm
    state fase1
      en:
      cube_operation=0100;
    state fase2
      en:
      cube_operation=0101;
    state fase3
      en:
      cube_operation=1101;
    state fase4
      en:
      cube_operation=1001;
    state fase6
      en:
      cube_operation=1100
    state fase8
      en:
      cube_operation=0110;
    state fase5
      en:
      cube_operation=1000;
    state fase7 %LMm
      en:
      cube_operation=1110;
    state fase9
      en:
      cube_operation=0100;
    state fase10
      en:
      cube_operation=1100;
    Ri.fase2 -> Ri.fase3 : [after(delay_ms,msec)]
    Ri.fase1 -> Ri.fase2 : [after(delay_ms,msec)]
    Ri.fase3 -> Ri.fase4 : [after(delay_ms,msec)]
    (default) -> Ri.fase1
    Ri.fase4 -> Ri.fase5 : [after(delay_ms,msec)]
    Ri.fase5 -> Ri.fase6 : [after(delay_ms,msec)]
    Ri.fase6 -> Ri.fase7 %LMm : [after(delay_ms,msec)]
    Ri.fase7 %LMm -> Ri.fase8 : [after(delay_ms,msec)]
    Ri.fase8 -> Ri.fase9 : [after(delay_ms,msec)]
    Ri.fase9 -> Ri.fase10 : [after(delay_ms,msec)]
  state Li
    en:
    %RTp
    %LMm
    state fase1
      en:
      cube_operation=1000;
    state fase2
      en:
      cube_operation=1001;
    state fase3
      en:
      cube_operation=1101;
    state fase4
      en:
      cube_operation=0101;
    state fase6
      en:
      cube_operation=1100
    state fase8
      en:
      cube_operation=0110;
    state fase7 %LMm
      en:
      cube_operation=1110;
    state fase5
      en:
      cube_operation=0100;
    state fase9
      en:
      cube_operation=0100;
    state fase10
      en:
      cube_operation=1100;
    Li.fase2 -> Li.fase3 : [after(delay_ms,msec)]
    Li.fase1 -> Li.fase2 : [after(delay_ms,msec)]
    Li.fase3 -> Li.fase4 : [after(delay_ms,msec)]
    (default) -> Li.fase1
    Li.fase4 -> Li.fase5 : [after(delay_ms,msec)]
    Li.fase6 -> Li.fase7 %LMm : [after(delay_ms,msec)]
    Li.fase5 -> Li.fase6 : [after(delay_ms,msec)]
    Li.fase7 %LMm -> Li.fase8 : [after(delay_ms,msec)]
    Li.fase8 -> Li.fase9 : [after(delay_ms,msec)]
    Li.fase9 -> Li.fase10 : [after(delay_ms,msec)]
  (default) -> wait_cube
  wait_cube -> webcam_alignment : [SW2==1 && SW2_status==0]
  webcam_alignment -> read_cube [order 2] : [SW3==1 && SW3_status==0]
  webcam_alignment -> wait_cube [order 1] : [SW2==1 && SW2_status==0]
  (junction 400) -> D [order 1] : [next_move(1)=='D' && next_move(2)==0]
  fase72 -> solve_cube : [SW3 == 1]
  D.fase4 -> (junction 752)
  (junction 735) -> Fi [order 1] : [next_move(1)=='F' && next_move(2)=='''']
  solve_cube -> (junction 747) : [execute_move == 1]
  (junction 774) -> solve_cube
  Fi.fase9 -> (junction 766)
  (junction 400) -> D2 [order 2] : [next_move(1)=='D' && next_move(2)=='2']
  (junction 747) -> (junction 400) [order 1]
  (junction 400) -> Di [order 3] : [next_move(1)=='D' && next_move(2)=='''']
  (junction 400) -> B [order 4] : [next_move(1)=='B' && next_move(2)==0]
  (junction 400) -> Bi [order 6] : [next_move(1)=='B' && next_move(2)=='''']
  (junction 400) -> B2 [order 5] : [next_move(1)=='B' && next_move(2)=='2']
  (junction 752) -> (junction 774)
  (junction 766) -> (junction 774)
  (junction 759) -> (junction 774)
  D2.fase7 -> (junction 752)
  (junction 735) -> F [order 2] : [[next_move(1)=='F' && next_move(2)==0]]
  Bi.fase4 -> (junction 752)
  Di.fase4 -> (junction 752)
  B.fase4 -> (junction 752)
  (junction 747) -> (junction 735) [order 2]
  B2.fase7 -> (junction 752)
  (junction 747) -> (junction 726) [order 3]
  F.fase9 -> (junction 766)
  F2.fase11 -> (junction 766)
  U2.fase16 -> (junction 766)
  U.fase13 -> (junction 766)
  (junction 735) -> F2 [order 3] : [next_move(1)=='F' && next_move(2)=='2']
  (junction 735) -> U [order 4] : [next_move(1)=='U' && next_move(2)==0]
  (junction 735) -> U2 [order 5] : [next_move(1)=='U' && next_move(2)=='2']
  (junction 726) -> Li [order 7] : [next_move(1)=='L' && next_move(2)=='''']
  (junction 726) -> Ui [order 2] : [next_move(1)=='U' && next_move(2)=='''']
  (junction 726) -> R [order 1] : [next_move(1)=='R' && next_move(2)==0]
  (junction 726) -> L2 [order 6] : [next_move(1)=='L' && next_move(2)=='2']
  (junction 726) -> R2 [order 3] : [[next_move(1)=='R' && next_move(2)=='2']]
  (junction 726) -> L [order 5] : [next_move(1)=='L' && next_move(2)==0]
  (junction 726) -> Ri [order 4] : [next_move(1)=='R' && next_move(2)=='''']
  R.fase10 -> (junction 759)
  R2.fase13 -> (junction 759)
  Ri.fase10 -> (junction 759)
  L.fase10 -> (junction 759)
  L2.fase13 -> (junction 759)
  Li.fase10 -> (junction 759)
  Ui.fase13 -> (junction 759)
  data: SW2 input; cube_operation output; SW3 input; SW3_status local =0; SW2_status local double =0; delay_ms constant double =3000; read_face output =0; webcam_alignment output =0; move_done output =1; read_done input; execute_move input; next_move data_store_memory
